simulink model "quadcopter_quaternions_rotatingAndBack2"  (R2023b)
settings: Solver=ode3  StartTime=0  StopTime=inf  FixedStep=0.005  RelTol=1e-3  EnableMultiTasking=on
values from neighbouring files (symbols this model uses):
  alpha_vect = A\B    [poly3traj.m]
  g = 9.81    [MRB.m]
  Ic = [Ixx,0,0;0,Iyy,0;0,0,Izz]    [MRB.m]
  m = 4    [MRB.m]
  Mrb = [m*eye(3),zeros(3);zeros(3),Ic]    [MRB.m]
libraries: aerolibutil x10, simulink_extras x9, slpidlib x6, sharedtransform x3, sharedutil x2, vrlib x2, dspsigops x1, dspmathops x1
(part 2 of 2)

== system quadcopter_quaternions_rotatingAndBack2/Formatting/Euler to VR/Quaternion Normalization ==
  e0 : Inport
  1/2 : Gain  Gain=1/2  SaturateOnIntegerOverflow=on  OutDataTypeStr=Inherit: Same as input  ParamDataTypeStr=Inherit: Same as input
  Demux : Demux  Outputs=[1 3]
      settings: DisplayOption=none
  Mux : Mux  Inputs=2
  Product : Product  InputSameDT=on  SaturateOnIntegerOverflow=on  OutDataTypeStr=Inherit: Same as first input
  Trigonometric Function : Trigonometry
  Trigonometric Function1 : Trigonometry  Operator=cos
  e0_norm : Outport  VectorParamsAs1DForOutWhenUnconnected=off
  wires:
  Trigonometric Function1/1 -> Mux/1
  Demux/2 -> Product/2
  Demux/1 -> 1/2/1
  Mux/1 -> e0_norm/1
  Product/1 -> Mux/2
  Trigonometric Function/1 -> Product/1
  1/2/1 -> Trigonometric Function1/1, Trigonometric Function/1
  e0/1 -> Demux/1

== system quadcopter_quaternions_rotatingAndBack2/Formatting/Euler to VR/Quaternion Normalization1 ==
  e0 : Inport
  1/2 : Gain  Gain=1/2  SaturateOnIntegerOverflow=on  OutDataTypeStr=Inherit: Same as input  ParamDataTypeStr=Inherit: Same as input
  Demux : Demux  Outputs=[1 3]
      settings: DisplayOption=none
  Mux : Mux  Inputs=2
  Product : Product  InputSameDT=on  SaturateOnIntegerOverflow=on  OutDataTypeStr=Inherit: Same as first input
  Trigonometric Function : Trigonometry
  Trigonometric Function1 : Trigonometry  Operator=cos
  e0_norm : Outport  VectorParamsAs1DForOutWhenUnconnected=off
  wires:
  e0/1 -> Demux/1
  1/2/1 -> Trigonometric Function/1, Trigonometric Function1/1
  Trigonometric Function/1 -> Product/1
  Product/1 -> Mux/2
  Mux/1 -> e0_norm/1
  Demux/1 -> 1/2/1
  Demux/2 -> Product/2
  Trigonometric Function1/1 -> Mux/1

== system quadcopter_quaternions_rotatingAndBack2/Formatting/Euler to VR/Quaternion Normalization2 ==
  e0 : Inport
  1/2 : Gain  Gain=1/2  SaturateOnIntegerOverflow=on  OutDataTypeStr=Inherit: Same as input  ParamDataTypeStr=Inherit: Same as input
  Demux : Demux  Outputs=[1 3]
      settings: DisplayOption=none
  Mux : Mux  Inputs=2
  Product : Product  InputSameDT=on  SaturateOnIntegerOverflow=on  OutDataTypeStr=Inherit: Same as first input
  Trigonometric Function : Trigonometry
  Trigonometric Function1 : Trigonometry  Operator=cos
  e0_norm : Outport  VectorParamsAs1DForOutWhenUnconnected=off
  wires:
  Trigonometric Function1/1 -> Mux/1
  Demux/2 -> Product/2
  Demux/1 -> 1/2/1
  Mux/1 -> e0_norm/1
  Product/1 -> Mux/2
  Trigonometric Function/1 -> Product/1
  1/2/1 -> Trigonometric Function1/1, Trigonometric Function/1
  e0/1 -> Demux/1

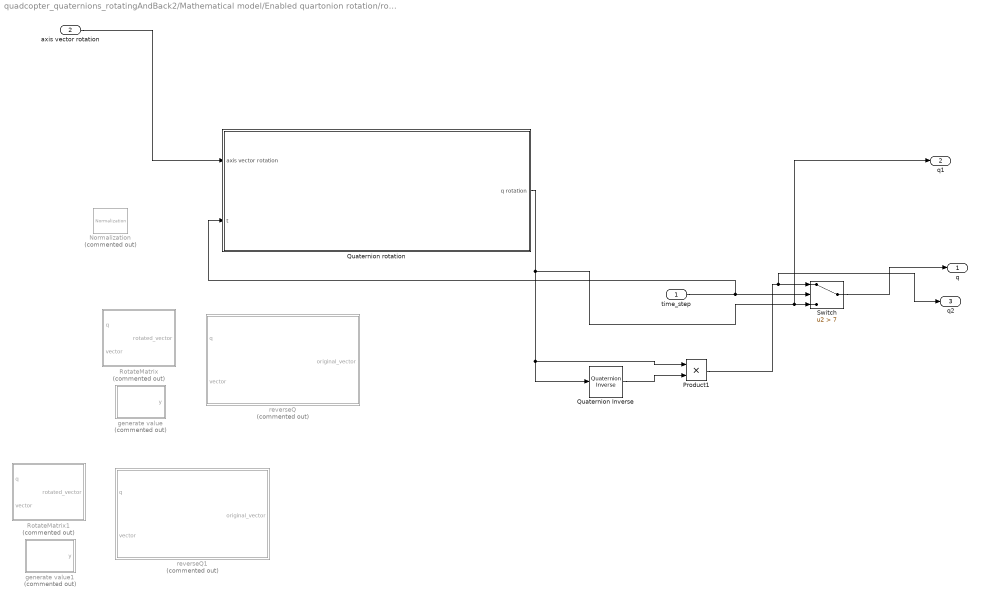
== system quadcopter_quaternions_rotatingAndBack2/Mathematical model/Enabled quartonion rotation/rotation system ==
  time_step : Inport
  axis vector rotation : Inport  Port=2
  Normalization : dspmathops/Normalization  Commented=on  NormType=Squared 2-norm  Bias=1e-10  NormOver=Each column  Dimension=1  roundingMode=Floor  overflowMode=off  accumDataTypeStr=Inherit: Same as product output  accumLastDataTypeStr=Inherit: Same as product output  outputDataTypeStr=Inherit: Same as product output  outputMin=[]  outputMax=[]  outputLastDataTypeStr=Inherit: Same as product output
  Product1 : Product
  Quaternion Inverse : aerolibutil/Quaternion Inverse
  "Quaternion rotation " : Subsystem
  RotateMatrix : MATLAB Function  Commented=on  TreatAsAtomicUnit=on
  RotateMatrix1 : MATLAB Function  Commented=on  TreatAsAtomicUnit=on
  Switch : Switch  Criteria=u2 > Threshold  Threshold=7  SaturateOnIntegerOverflow=off  InputSameDT=off
  generate value : MATLAB Function  Commented=on  TreatAsAtomicUnit=on
  generate value1 : MATLAB Function  Commented=on  TreatAsAtomicUnit=on
  reverseQ : MATLAB Function  Commented=on  TreatAsAtomicUnit=on
  reverseQ1 : MATLAB Function  Commented=on  TreatAsAtomicUnit=on
  q : Outport
  q1 : Outport  Port=2
  q2 : Outport  Port=3
  wires:
  "Quaternion rotation "/1(q rotation) -> Product1/1, Quaternion Inverse/1, q1/1, Switch/3
  Switch/1 -> q/1
  Product1/1 -> q2/1, Switch/1
  time_step/1 -> Switch/2, "Quaternion rotation "/2(t)
  Quaternion Inverse/1 -> Product1/2
  axis vector rotation/1 -> "Quaternion rotation "/1(axis vector rotation)

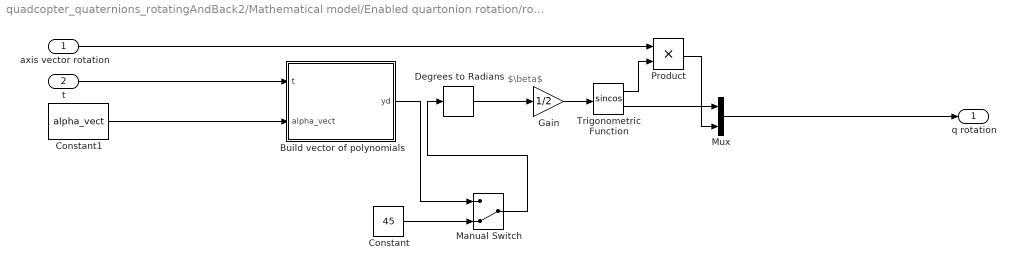
== system quadcopter_quaternions_rotatingAndBack2/Mathematical model/Enabled quartonion rotation/rotation system/Quaternion rotation  ==
  note: $\beta$
  axis vector rotation : Inport
  t : Inport  Port=2
  Build vector of polynomials : MATLAB Function  TreatAsAtomicUnit=on
  Constant : Constant  Value=45
  Constant1 : Constant  Value=alpha_vect  VectorParams1D=off
  Degrees to Radians : simulink_extras/Transformations/Degrees to Radians
  Gain : Gain  Gain=1/2
  Manual Switch : ManualSwitch  CurrentSetting=0
  Mux : Mux  Inputs=2
  Product : Product
  Trigonometric Function : Trigonometry  Operator=sincos
  q rotation : Outport
  wires:
  Gain/1 -> Trigonometric Function/1
  Trigonometric Function/2 -> Mux/1
  axis vector rotation/1 -> Product/1
  Degrees to Radians/1 -> Gain/1
  Trigonometric Function/1 -> Product/2
  Constant1/1 -> Build vector of polynomials/2(alpha_vect)
  Product/1 -> Mux/2
  Mux/1 -> q rotation/1
  Build vector of polynomials/1(yd) -> Manual Switch/1
  Manual Switch/1 -> Degrees to Radians/1
  t/1 -> Build vector of polynomials/1(t)
  Constant/1 -> Manual Switch/2

== matlab function quadcopter_quaternions_rotatingAndBack2/Mathematical model/scaled time 2 ==
  data: t1 input; counter_timer input; t2 output; counter_timer output
function [t2, counter_timer] = fcn(t1,counter_timer)
 
if t1 == counter_timer(2)
   counter_timer(1) = counter_timer(1) +1; 
   counter_timer(2) = counter_timer(2) + 2.5;
      
end
if counter_timer(1) == 11
  counter_timer(1) = 0;
end

t2 = counter_timer(1);

== matlab function quadcopter_quaternions_rotatingAndBack2/Flight Control System/Outer loop position control/MATLAB Function ==
  data: Deltap_e input; Deltap_b output; psi input
function Deltap_b = fcn(Deltap_e,psi)

R = [ cos(psi) , -sin(psi) ;
      sin(psi) ,  cos(psi) ];

Deltap_b = R'*Deltap_e;

== matlab function quadcopter_quaternions_rotatingAndBack2/Mathematical model/ memory hold block ==
  data: q input; q_forward input; q_inverse input; q2 output; prev_q input; prev_q output
function [q2,prev_q] = fcn(q,q_forward,q_inverse,prev_q)
dq = floor(q(1)*10000);% represenation of q1 as a 4 digit number
prev_dq = floor(prev_q(1)*10000); % previous q1
if q ==  [0; 0; 0; 0] 
    q = [1 ;0; 0; 0];
end
disp(q);

if dq ==  floor(q_inverse(1)*10000)
 q = [1 ;0; 0; 0];
 prev_q = q(1);
end

if dq == floor(q_forward(1)*10000) && prev_dq ==  floor(q_inverse(1)*10000) % 45 degree back and forth indicators represented at a whole numbers of the first element quartonion value. 

  q = [1 ;0; 0; 0];
  prev_q = q(1);

end
q2 = q;

== matlab function quadcopter_quaternions_rotatingAndBack2/Mathematical model/Enabled quartonion rotation/rotation system/RotateMatrix ==
  data: q input; rotated_vector output; vector input
function rotated_vector = applyQuaternionRotation(q, vector)
    % quaternion components
    w = q(1);
    x = q(2);
    y = q(3);
    z = q(4);
    % Quaternion rotation matrix
    R = [1 - 2*y^2 - 2*z^2, 2*x*y - 2*z*w, 2*x*z + 2*y*w;
         2*x*y + 2*z*w, 1 - 2*x^2 - 2*z^2, 2*y*z - 2*x*w;
         2*x*z - 2*y*w, 2*y*z + 2*x*w, 1 - 2*x^2 - 2*y^2];
    % rotate
    rotated_vector = R * vector;
end

== matlab function quadcopter_quaternions_rotatingAndBack2/Build vector of polynomials ==
  data: t input; yd output; alpha_vect input
function yd = fcn(t,alpha_vect)

    %t_vect0 = [ 1 ; t ; t^2 ; t^3 ; t^4 ; t^5 ]; % vector of t values
    t_vect0 = [1; t; t^2; t^3];  % vector of t values for cubic polynomial
 
yd = t_vect0'*alpha_vect;

== matlab function quadcopter_quaternions_rotatingAndBack2/Mathematical model/Enabled quartonion rotation/rotation system/Quaternion rotation /Build vector of polynomials ==
  data: t input; yd output; alpha_vect input
function yd = fcn(t,alpha_vect)


    t_vect0 = [ 1 ; t ; t^2 ; t^3 ; t^4 ; t^5 ]; % vector of t values
    %t_vect0 = [ 1 ; t ; t^2 ; t^3 ]; % vector of t values


yd = t_vect0'*alpha_vect;

== matlab function quadcopter_quaternions_rotatingAndBack2/Mathematical model/Rigid-body dynamics1/MATLAB Function ==
  data: nu input; Cnunu output; m input; Ic input
function Cnunu = fcn(nu,m,Ic)

v = nu(1:3);  % linear velocities (expressed in the body frame)
omega = nu(4:6); % angular velocities (expressed in the body frame)

% Coriolis term
Cnunu = [ cross(omega,m*v) ; -cross(Ic*omega,omega) ];

== matlab function quadcopter_quaternions_rotatingAndBack2/Mathematical model/Enabled quartonion rotation/rotation system/generate value ==
  data: y output
function y = random_counter()
    persistent counter;
    
    % Initialize counter if not already initialized
    if isempty(counter)
        counter = 0;
    end
    
    % Increment counter
    counter = counter + 1;
    display(counter)
    % Check if counter has reached a random interval between 0 and 20
    if counter >= 2
        
        % Reset counter to 0
        counter = 0;
    end
    
    y = counter;
end

== matlab function quadcopter_quaternions_rotatingAndBack2/Mathematical model/Enabled quartonion rotation/rotation system/reverseQ ==
  data: q input; original_vector output; vector input
function original_vector = revertQuaternionRotation(q, vector)
    % Extract quaternion components
    w = q(1);
    x = -q(2);
    y = -q(3);
    z = -q(4);
    % Inverse quaternion (conjugate for unit quaternion)
    % Apply inverse rotation
     % Quaternion rotation matrix again but with the inverse quartonion
     % this time
    R = [1 - 2*y^2 - 2*z^2, 2*x*y - 2*z*w, 2*x*z + 2*y*w;
         2*x*y + 2*z*w, 1 - 2*x^2 - 2*z^2, 2*y*z - 2*x*w;
         2*x*z - 2*y*w, 2*y*z + 2*x*w, 1 - 2*x^2 - 2*y^2];
    % Apply rotation on the inverse
    original_vector = R * vector;
end

== matlab function quadcopter_quaternions_rotatingAndBack2/Mathematical model/Enabled quartonion rotation/rotation system/RotateMatrix1 ==
  data: q input; rotated_vector output; vector input
function rotated_vector = applyQuaternionRotation(q, vector)
    % quaternion components
    w = q(1);
    x = q(2);
    y = q(3);
    z = q(4);
    % Quaternion rotation matrix
    R = [1 - 2*y^2 - 2*z^2, 2*x*y - 2*z*w, 2*x*z + 2*y*w;
         2*x*y + 2*z*w, 1 - 2*x^2 - 2*z^2, 2*y*z - 2*x*w;
         2*x*z - 2*y*w, 2*y*z + 2*x*w, 1 - 2*x^2 - 2*y^2];
    % rotate
    rotated_vector = R * vector;
end

== matlab function quadcopter_quaternions_rotatingAndBack2/Mathematical model/Enabled quartonion rotation/rotation system/generate value1 ==
  data: y output
function y = random_counter()
    persistent counter;
    
    % Initialize counter if not already initialized
    if isempty(counter)
        counter = 0;
    end
    
    % Increment counter
    counter = counter + 1;
    display(counter)
    % Check if counter has reached a random interval between 0 and 20
    if counter >= 2
        
        % Reset counter to 0
        counter = 0;
    end
    
    y = counter;
end

== matlab function quadcopter_quaternions_rotatingAndBack2/Mathematical model/Enabled quartonion rotation/rotation system/reverseQ1 ==
  data: q input; original_vector output; vector input
function original_vector = revertQuaternionRotation(q, vector)
    % Extract quaternion components
    w = q(1);
    x = -q(2);
    y = -q(3);
    z = -q(4);
    % Inverse quaternion (conjugate for unit quaternion)
    % Apply inverse rotation
     % Quaternion rotation matrix again but with the inverse quartonion
     % this time
    R = [1 - 2*y^2 - 2*z^2, 2*x*y - 2*z*w, 2*x*z + 2*y*w;
         2*x*y + 2*z*w, 1 - 2*x^2 - 2*z^2, 2*y*z - 2*x*w;
         2*x*z - 2*y*w, 2*y*z + 2*x*w, 1 - 2*x^2 - 2*y^2];
    % Apply rotation on the inverse
    original_vector = R * vector;
end
